simulink model "generated_signal"  (R2016b)
settings: Solver=VariableStepAuto  StartTime=0.0  StopTime=10.0  RelTol=1e-3
undefined symbols (not defined in the file): sigbuilder_block
libraries: fuzblock x1
settings Model: Creator=ASUS  LastModifiedBy=ASUS

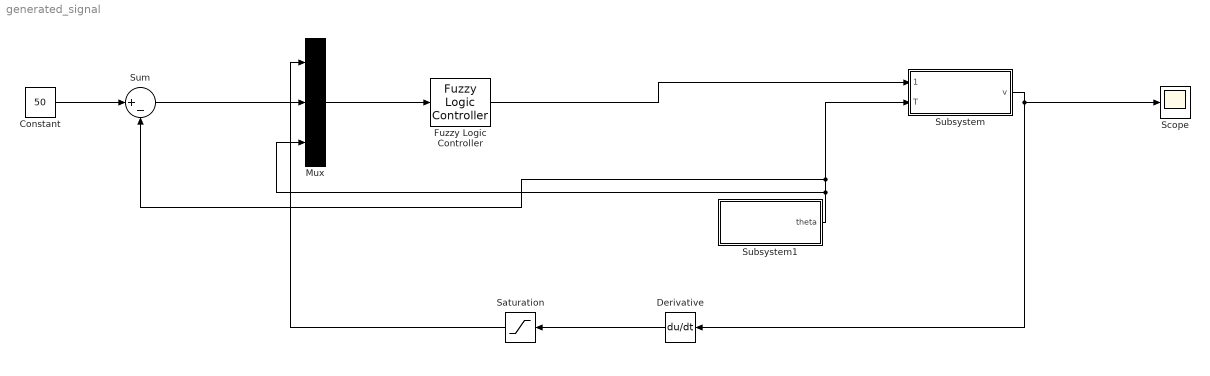
== system generated_signal ==
  Constant : Constant  Value=50
  Derivative : Derivative
  Fuzzy Logic Controller : fuzblock/Fuzzy Logic  Controller  fis=[]
  Mux : Mux  Inputs=3
  Saturation : Saturate
  Scope : Scope
  Subsystem : Subsystem
  Subsystem1 : Subsystem
  Sum : Sum  Inputs=|+-
  wires:
  Mux/1 -> Fuzzy Logic Controller/1
  Subsystem/1(v) -> Scope/1, Derivative/1
  Derivative/1 -> Saturation/1
  Saturation/1 -> Mux/1
  Sum/1 -> Mux/2
  Constant/1 -> Sum/1
  Subsystem1/1(theta) -> Mux/3, Sum/2, Subsystem/2(T)
  Fuzzy Logic Controller/1 -> Subsystem/1

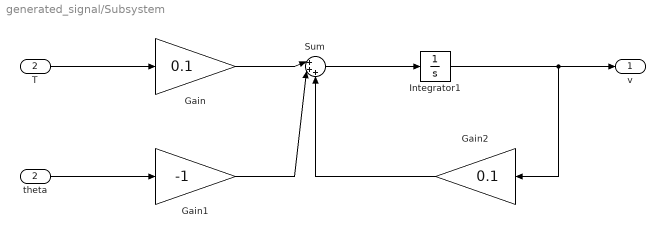
== system generated_signal/Subsystem ==
  T : Inport  Port=2
  Gain : Gain  Gain=0.1
  Gain1 : Gain  Gain=-1
  Gain2 : Gain  Gain=0.1
  Integrator1 : Integrator
  Sum : Sum  Inputs=|+++
  theta : InportShadow  Port=2
  v : Outport
  wires:
  T/1 -> Gain/1
  theta/1 -> Gain1/1
  Gain1/1 -> Sum/2
  Gain/1 -> Sum/1
  Gain2/1 -> Sum/3
  Integrator1/1 -> Gain2/1, v/1
  Sum/1 -> Integrator1/1

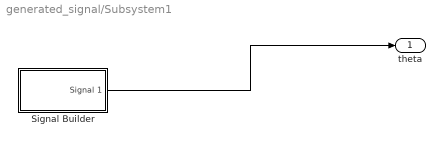
== system generated_signal/Subsystem1 ==
  Signal Builder : Subsystem  Tag=STV Subsys  LoadFcn=sigbuilder_block('load');  StartFcn=sigbuilder_block('start');  StopFcn=sigbuilder_block('stop');  ClipboardFcn=sigbuilder_block('clipboard');  mask(Sigbuilder block){tuvar=[0:10]}
      mask help: Simulink:masks:SigbuilderBlock_MD
      mask init:
      | if ~strcmp(get_param(bdroot(gcbh),'SimulationStatus'),'stopped') tuvar = sigbuilder_block('maskInit'); end
      settings: CopyFcn=sigbuilder_block('copy');  DeleteFcn=sigbuilder_block('delete');  ModelCloseFcn=sigbuilder_block('modelClose');  PreSaveFcn=sigbuilder_block('preSave');  PauseFcn=sigbuilder_block('pause');  ContinueFcn=sigbuilder_block('continue');  NameChangeFcn=sigbuilder_block('namechange');  OpenFcn=sigbuilder_block('open',[265.2 145.8 550.8 400.2 ]);  CloseFcn=sigbuilder_block('close');
      mask Display: plot(0, 0, 100, 100,[2, 2, 32, 32, 2], [68, 8, 8, 68, 68],[32, 2], [38, 38], [32, 19, 2],[53, 60, 44], [32, 17, 17, 2],[16, 16, 31, 31]);txt = getActiveGroup(gcbh);text(2, 100, txt,'verticalAlignment', 'top');
  theta : Outport
  wires:
  Signal Builder/1(Signal 1) -> theta/1

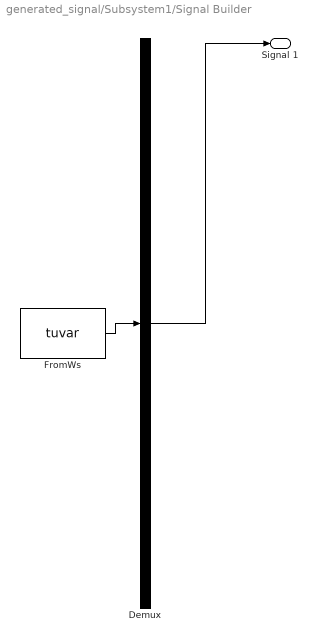
== system generated_signal/Subsystem1/Signal Builder ==
  Demux : Demux  Tag=STV Demux  Outputs=1
  FromWs : FromWorkspace  Tag=STV FromWs  VariableName=tuvar  SampleTime=0
      SigBuilderData=|
      | common.afterFinalStr = 'Extrapolate'
      | common.sampleTime = 0
      | dataSet.timeRange = [0 100]
      | dataSet.name = 'Group 1'
      | sbobj.Groups.Name = 'Group 1'
      | sbobj.Groups.Signals.Name = 'Signal 1'
      | sbobj.Groups.Signals.XData = [0 20 40 80 100]
      | sbobj.Groups.Signals.YData = [-5 0 0 10 10]
      | sbobj.Groups.TimeRange = [0 100]
  Signal 1 : Outport  Tag=STV Outport
  wires:
  Demux/1 -> Signal 1/1
  FromWs/1 -> Demux/1
